simulink model "ALGO_TrajTrack_Qband"  (R2023a)
settings: Solver=VariableStepAuto  StartTime=0.0  StopTime=60  RelTol=1e-3
StopFcn:
  | CompareSimResult_anti_rollover
libraries: simulink x7, slpidlib x1, Solver_SF x1
(part 1 of 2)
CloseFcn:
  | sp_simResult_save
settings Model: Creator=QXJ  LastModifiedBy=28303
settings SolverCC: AlgebraicLoopSolver=TrustRegion
settings DebuggingCC: UnconnectedInputMsg=warning  UnconnectedOutputMsg=warning  UnconnectedLineMsg=warning
settings ModelReferenceCC: EnableRefExpFcnMdlSchedulingChecks=on
settings SFSimCC: CustomCodeUndefinedFunction=UseInterfaceOnly

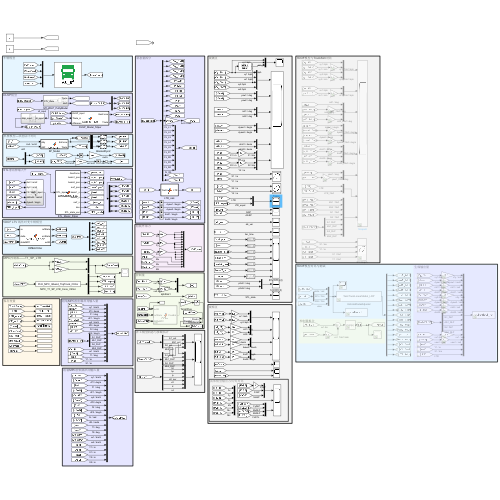
[thumbnail: Simulink's stored preview of the top-level diagram]
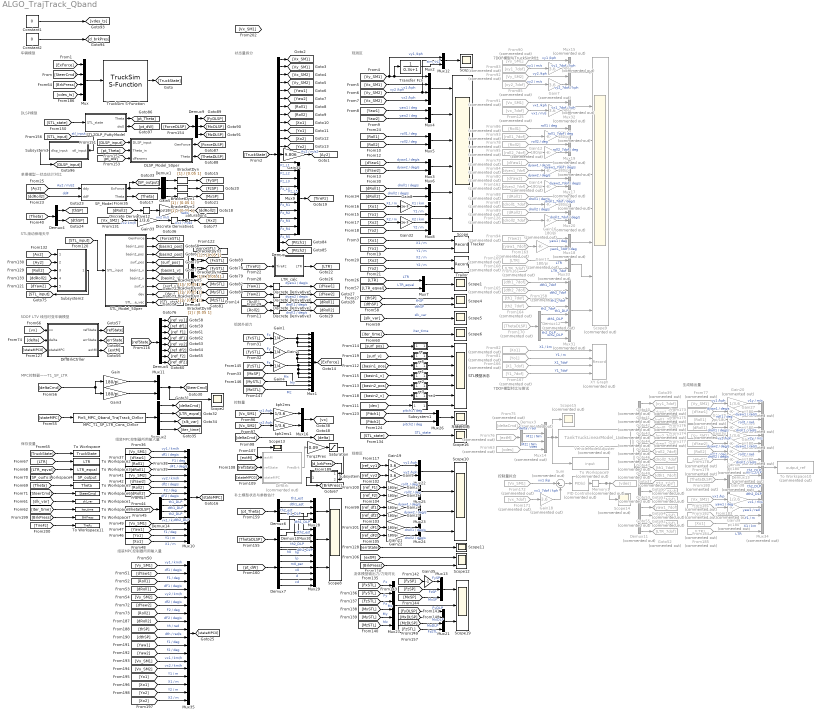
== system ALGO_TrajTrack_Qband ==
  note: 7DOF模型对比与测试
  note: 生成输出量
  note: 控制量拟合
  note: 7DOF模型与TruckSim对比
  note: 补土模型状态与参数估计
  note: 流体模型输出力/力矩对比
  note: MPC控制器——T1_SP_LTR
  note: 组装MPC控制器所用输入量
  note: 观测区
  note: 车辆模型
  note: 组装外部力
  note: 单摆模型---状态估计对比
  note: 状态量拆分
  note: 保存变量
  note: 5DOF LTV 线性时变车辆模型
  note: 观察区
  note: 控制量
  note: STL滑动伸缩天平
  note: DLSP模型
  note: 组装MPC控制器所用输入量
  BracketDyn{,1..8} (9 alike) : TransferFcn  Denominator=[0.05 1]
  Constant1 : Constant  Value=0
  Constant2 : Constant  Value=0
  DLSP_Model_50per : MATLAB Function  TreatAsAtomicUnit=on  SystemSampleTime=0.01
  Demux : Demux  Outputs=25
  Demux1 : Demux  Outputs=3
  Demux{2,6,10,14} (4 alike) : Demux
  Demux11 : Demux  Commented=on  Outputs=17
  Demux12 : Demux  Commented=on
  Demux13 : Demux  Commented=on
  Demux3 : Demux  Commented=on  Outputs=2
  Demux4 : Demux  Outputs=2
  Demux5 : Demux  Outputs=8
  Demux7 : Demux  Outputs=7
  Demux8 : Demux  Outputs=6
  Demux9 : Demux  Outputs=3
  DiffBrk : MATLAB Function  Commented=on  TreatAsAtomicUnit=on
  DiffBrkCtrller : MATLAB Function  TreatAsAtomicUnit=on  SystemSampleTime=0.01
  Discrete Derivative1 : simulink/Discrete/Discrete Derivative  gainval=1.0  ICPrevScaledInput=0  OutMin=[-9.806*0.6]  OutMax=[9.806*0.6]  OutDataType=fixdt(1, 16)  OutScaling=2^-10  DoSatur=off
  Discrete Derivative{2..3,5..6,12} (5 alike) : simulink/Discrete/Discrete Derivative  gainval=1.0  ICPrevScaledInput=0.0  OutMin=[]  OutMax=[]  OutDataType=fixdt(1, 16)  OutScaling=2^-10  DoSatur=off
  From125 : From  Commented=on  GotoTag=vx_7dof
  From126 : From  Commented=on  GotoTag=droll2_7dof
  From158 : From  Commented=on  GotoTag=th1_7dof
  From161 : From  Commented=on  GotoTag=dth1_7dof
  From162 : From  Commented=on  GotoTag=dyaw2_7dof
  From163 : From  Commented=on  GotoTag=yaw1_7dof
  From164 : From  Commented=on  GotoTag=th2_7dof
  From165 : From  Commented=on  GotoTag=dth2_7dof
  From166 : From  Commented=on  GotoTag=X1_7dof
  From167 : From  Commented=on  GotoTag=Y1_7dof
  From168 : From  Commented=on  GotoTag=LTR_7dof
  From169 : From  Commented=on  GotoTag=LTR
  From170 : From  Commented=on  GotoTag=ThetaDLSP
  From171 : From  Commented=on  GotoTag=vx_7dof
  From172 : From  Commented=on  GotoTag=Vx_SM1
  From173 : From  Commented=on  GotoTag=dYaw1
  From174 : From  Commented=on  GotoTag=Vy_SM2
  From175 : From  Commented=on  GotoTag=Roll1
  From176 : From  Commented=on  GotoTag=dRoll1
  From177 : From  Commented=on  GotoTag=dYaw2
  From178 : From  Commented=on  GotoTag=Roll2
  From179 : From  Commented=on  GotoTag=dRoll2
  From180 : From  Commented=on  GotoTag=ThetaDLSP
  From181 : From  Commented=on  GotoTag=Vx_SM1
  From182 : From  Commented=on  GotoTag=Yaw1
  From183 : From  Commented=on  GotoTag=Yo1
  From184 : From  Commented=on  GotoTag=Xo1
  From185 : From  Commented=on  GotoTag=LTR
  From63 : From  Commented=on  GotoTag=vdes
  From75 : From  Commented=on  GotoTag=deltaCmd
  From76 : From  Commented=on  GotoTag=extM
  From77 : From  Commented=on  GotoTag=Vy_SM1
  From78 : From  Commented=on  GotoTag=Roll2
  From79 : From  Commented=on  GotoTag=dYaw1
  From80 : From  Commented=on  GotoTag=dYaw2
  From81 : From  Commented=on  GotoTag=Yo1
  From82 : From  Commented=on  GotoTag=Xo1
  From83 : From  Commented=on  GotoTag=vy1_7dof
  From84 : From  Commented=on  GotoTag=dyaw1_7dof
  From85 : From  Commented=on  GotoTag=vy2_7dof
  From86 : From  Commented=on  GotoTag=Roll1
  From87 : From  Commented=on  GotoTag=droll1_7dof
  From88 : From  Commented=on  GotoTag=dRoll1
  From89 : From  Commented=on  GotoTag=dRoll2
  From90 : From  Commented=on  GotoTag=Vy_SM1
  From91 : From  Commented=on  GotoTag=Vx_SM1
  From92 : From  Commented=on  GotoTag=Vy_SM2
  From93 : From  Commented=on  GotoTag=roll1_7dof
  From94 : From  Commented=on  GotoTag=Yaw1
  From95 : From  Commented=on  GotoTag=roll2_7dof
  Gain{,3,21..26} (8 alike) : Gain  Gain=180/pi
  Gain1 : Gain  Gain=1/4
  Gain{6..7,10,18} (4 alike) : Gain  Commented=on  Gain=3.6
  Gain{11..17} (7 alike) : Gain  Commented=on  Gain=180/pi
  Gain19 : Gain  Gain=3.6
  Gain2 : Gain  Gain=1/4
  Gain20 : Gain  Commented=on  Gain=1/3.6
  Gain{27..29,31,36..37,39} (7 alike) : Gain  Commented=on  Gain=pi/180
  Gain30 : Gain  Commented=on  Gain=1/3.6
  Gain32 : Gain  Gain=1e-3
  Gain33 : Gain  Gain=1/3.6
  Gain34 : Gain  Gain=9.806
  Gain35 : Gain  Gain=-1
  Gain38 : Gain  Commented=on  Gain=1/3.6
  Gain4 : Gain  Gain=1/4
  Gain5 : Gain  Gain=pi/180
  Gain8 : Gain  Gain=1e-3
  Gain9 : Gain  Gain=3.6
  Goto37 : Goto  Commented=on  GotoTag=vdes
  Goto39 : Goto  Commented=on  GotoTag=vy1_7dof
  Goto40 : Goto  Commented=on  GotoTag=dyaw1_7dof
  Goto41 : Goto  Commented=on  GotoTag=roll1_7dof
  Goto42 : Goto  Commented=on  GotoTag=droll1_7dof
  Goto43 : Goto  Commented=on  GotoTag=vy2_7dof
  Goto44 : Goto  Commented=on  GotoTag=dyaw2_7dof
  Goto45 : Goto  Commented=on  GotoTag=roll2_7dof
  Goto46 : Goto  Commented=on  GotoTag=droll2_7dof
  Goto47 : Goto  Commented=on  GotoTag=th1_7dof
  Goto49 : Goto  Commented=on  GotoTag=dth1_7dof
  Goto50 : Goto  Commented=on  GotoTag=th2_7dof
  Goto51 : Goto  Commented=on  GotoTag=dth2_7dof
  Goto52 : Goto  Commented=on  GotoTag=LTR_7dof
  Goto53 : Goto  Commented=on  GotoTag=vx_7dof
  Goto54 : Goto  Commented=on  GotoTag=yaw1_7dof
  Goto55 : Goto  Commented=on  GotoTag=X1_7dof
  Goto92 : Goto  Commented=on  GotoTag=Y1_7dof
  "LTR_calc " : MATLAB Function  TreatAsAtomicUnit=on
  MPC_T1_SP_LTR_Cons_Ctrllor : S-Function  FunctionName=Pin5_MPC_Qband_TrajTrack_Ctrllor  SFunctionDeploymentMode=off  EnableBusSupport=off
  Memory1 : Memory  Commented=on  InitialCondition=70/3.6
  Mux{,2,8,21,28,30} (6 alike) : Mux
  Mux1 : Mux  Inputs=15
  Mux10 : Mux  Inputs=16
  Mux{3..7,11,16,22..26} (12 alike) : Mux  Inputs=2
  Mux12 : Mux  Inputs=3
  Mux13 : Mux  Inputs=3
  Mux{14..15,17,19..20} (5 alike) : Mux  Commented=on
  Mux18 : Mux  Commented=on  Inputs=2
  Mux27 : Mux  Inputs=6
  Mux29 : Mux  Inputs=7
  Mux31 : Mux  Commented=on  Inputs=8
  Mux32 : Mux  Commented=on  Inputs=2
  Mux33 : Mux  Commented=on  Inputs=2
  Mux34 : Mux  Commented=on  Inputs=17
  Mux35 : Mux  Inputs=18
  Mux9 : Mux  Inputs=10
  PID Controller : slpidlib/PID Controller  Commented=on  Controller=PID  Form=Parallel  TimeDomain=Continuous-time  UseExternalTs=off  SampleTime=-1  IntegratorMethod=Forward Euler  FilterMethod=Forward Euler  ControllerParametersSource=internal  P=5  I=5  UseKiTs=off  D=0  N=100  UseFilter=on  TunerSelectOption=Transfer Function Based (PID Tuner App)  InitialConditionSource=internal  InitialConditionForIntegrator=20  InitialConditionForFilter=0  DifferentiatorICPrevScaledInput=0  ExternalReset=none  TrackingMode=off  Kt=1  LimitOutput=off  SatLimitsSource=internal  UpperSaturationLimit=inf  LowerSaturationLimit=-inf  LinearizeAsGain=on  AntiWindupMode=none  Kb=1  LimitIntegrator=off  UpperIntegratorSaturationLimit=inf  LowerIntegratorSaturationLimit=-inf  POutMin=[]  POutMax=[]  IOutMin=[]  IOutMax=[]  DOutMin=[]  DOutMax=[]  NOutMin=[]  NOutMax=[]  SumOutMin=[]  SumOutMax=[]  SaturationOutMin=[]  SaturationOutMax=[]  PParamMin=[]  PParamMax=[]  IParamMin=[]  IParamMax=[]  DParamMin=[]  DParamMax=[]  NParamMin=[]  NParamMax=[]  KbParamMin=[]  KbParamMax=[]  KtParamMin=[]  KtParamMax=[]  KbOutMin=[]  KbOutMax=[]  KtOutMin=[]  KtOutMax=[]  IntegratorOutMin=[]  IntegratorOutMax=[]  FilterOutMin=[]  FilterOutMax=[]  SumI1OutMin=[]  SumI1OutMax=[]  SumI2OutMin=[]  SumI2OutMax=[]  SumI3OutMin=[]  SumI3OutMax=[]  SumI4OutMin=[]  SumI4OutMax=[]  SumDOutMin=[]  SumDOutMax=[]  DifferentiatorOutMin=[]  DifferentiatorOutMax=[]  FilterDiffOutCoefMin=[]  FilterDiffOutCoefMax=[]  ReciprocalOutMin=[]  ReciprocalOutMax=[]  SumDenOutMin=[]  SumDenOutMax=[]  SumNumOutMin=[]  SumNumOutMax=[]  DivideOutMin=[]  DivideOutMax=[]  UdiffTsProdOutMin=[]  UdiffTsProdOutMax=[]  NTsProdOutMin=[]  NTsProdOutMax=[]  UintegralTsProdOutMin=[]  UintegralTsProdOutMax=[]  UngainTsProdOutMin=[]  UngainTsProdOutMax=[]  ClampingZeroOutDataTypeStr=Inherit: Inherit via back propagation  ClampingZeroOutMin=[]  ClampingZeroOutMax=[]  FilterDenConstantOutDataTypeStr=Inherit: Inherit via back propagation  FilterDenConstantOutMin=[]  FilterDenConstantOutMax=[]  PCopyOutDataTypeStr=Inherit: Inherit via back propagation  PCopyOutMin=[]  PCopyOutMax=[]  NCopyOutDataTypeStr=Inherit: Inherit via back propagation  NCopyOutMin=[]  NCopyOutMax=[]  IntegratorContinuousStateAttributes=''  IntegratorStateMustResolveToSignalObject=off  IntegratorRTWStateStorageClass=Auto  FilterContinuousStateAttributes=''  FilterStateMustResolveToSignalObject=off  FilterRTWStateStorageClass=Auto  ParallelPVariant=InternalParameters  IdealPVariant=Disabled  IVariant=InternalParameters  DVariant=InternalParameters  IntegratorVariant=Continuous  SatVariant=Disabled  AWVariant=Passthrough  PCopyVariant=Disabled  TRVariant=Disabled  FdbkBlocksVariant=Forward  IdealPFdbkVariant=Disabled  SatFdbkVariant=Disabled  DerivativeFilterVariant=ContFilter  NVariant=InternalParameters  NCopyVariant=Disabled  FilterICVariant=InternalICsFilter  IntegratorICVariant=InternalICs  ExternalResetVariant=Disabled  TRSumVariant=Passthrough  SumFdbkVariant=Disabled  SumVariant=Sum_PID  TsampFilterVariant=InternalTs  TsampNgainVariant=Passthrough  TsampIntegralVariant=Disabled_SignalSpec  ExternalSaturationOutDataTypeStr=Inherit: Same as second input
  SP_Model : MATLAB Function  TreatAsAtomicUnit=on  SystemSampleTime=0.005
  STL2DLP_PuttyModel : Subsystem
  STL_Model_50per : MATLAB Function  TreatAsAtomicUnit=on  SystemSampleTime=0.01
  STL模型状态 : Scope  NumInputPorts=7
  Saturation : Saturate  UpperLimit=0.75  LowerLimit=0
  Saturation1 : Saturate  UpperLimit=9.806*0.6  LowerLimit=-9.806*0.6
  Scope : Scope  NumInputPorts=6
  Scope{1..3,5..6,11,13,16} (8 alike) : Scope
  Scope10 : Scope  NumInputPorts=4
  Scope12 : Scope  NumInputPorts=2
  Scope14 : Scope  Commented=on
  Scope15 : Scope  Commented=on
  Scope19 : Scope  NumInputPorts=3
  Scope4 : Scope  NumInputPorts=2
  Scope8 : Scope  NumInputPorts=3
  Scope9 : Scope  Commented=on  NumInputPorts=8
  Subsystem : Subsystem
  Subsystem1 : Subsystem
  Subsystem2 : Subsystem
  Subsystem3 : Subsystem
  Sum : Sum  Commented=on  Inputs=|+-
  To Workspace : ToWorkspace  VariableName=TruckState  SaveFormat=Timeseries  SampleTime=-1
  To Workspace1 : ToWorkspace  VariableName=skl_var  SaveFormat=Timeseries  SampleTime=-1
  To Workspace10 : ToWorkspace  Commented=on  VariableName=output_ref  SaveFormat=Timeseries  SampleTime=-1
  To Workspace11 : ToWorkspace  VariableName=TireFz  SaveFormat=Timeseries  SampleTime=-1
  To Workspace2 : ToWorkspace  VariableName=LTR  SaveFormat=Timeseries  SampleTime=-1
  To Workspace3 : ToWorkspace  VariableName=LTR_eqval  SaveFormat=Timeseries  SampleTime=-1
  To Workspace4 : ToWorkspace  VariableName=SP_output  SaveFormat=Timeseries  SampleTime=-1
  To Workspace5 : ToWorkspace  VariableName=Theta  SaveFormat=Timeseries  SampleTime=-1
  To Workspace6 : ToWorkspace  VariableName=SteerCmd  SaveFormat=Timeseries  SampleTime=-1
  To Workspace7 : ToWorkspace  VariableName=BrkPress  SaveFormat=Timeseries  SampleTime=-1
  To Workspace8 : ToWorkspace  VariableName=iter_time  SaveFormat=Timeseries  SampleTime=-1
  To Workspace9 : ToWorkspace  Commented=on  VariableName=input  SaveFormat=Timeseries  SampleTime=-1
  Torq2Pres : Gain  Gain=0.09
  Tracker : Record  FileSettingsInternal="{\"entries\":[{\"content\":{\"excelSettings\":{\"content\":{},\"type\":\"Streamout.ExcelSettings\"}},\"type\":\"Streamout.FileSettingStorage\",\"uuid\":\"10e10eac-3b42-48c4-b005-3ff0f1f86fec\"}],\"packageUris\":[\"http://schema.mathworks.com/mf0/streamout_blocks/R2020a\"],\"version\":\"1.0\"}"  Layout=[1 1]  SignalsInternal="{\"entries\":[{\"content\":{\"signals\":[{\"content\":{\"blockPath\":[\"ALGO_TrajTrack_Qband/Tracker\"],\"dimensions\":[1],\"domain\":\"ALGO_TrajTrack_Qband/Tracker\",\"lineColor\":\"#64d413\",\"port\":1,\"sid\":[\"\"],\"signalID\":23696,\"signalName\":\"X1 / m\"},\"type\":\"RecordBlkView.Signal\",\"uuid\":\"81066948-288f-4e97-bbd3-45679b52fbb6\"},{\"content\":{\"blockPath\":[\"ALGO_TrajTrack_Qband/Tracker\"],\"dimensions\":[1],\"domain\":\"ALGO_TrajTrack_Qband/Tracker\",\"lineColor\":\"#ff13a6\",\"port\":2,\"sid\":[\"\"],\"signalID\":23700,\"signalName\":\"Y1 / m\"},\"type\":\"RecordBlkView.Signal\",\"uuid\":\"ec9d7904-73b7-4926-97ce-8ccb334fc86a\"}]},\"type\":\"RecordBlkView.InputSignals\",\"uuid\":\"48fa4a27-7477-4a7c-bc50-316526f17c74\"}],\"packageUris\":[\"http://schema.mathworks.com/mf0/streamout_blocks/R2020a\"],\"version\":\"1.0\"}"  VisualizationBindings="{\"xyplotplugin\":{\"info\":[{\"series\":[],\"subplotID\":1}]}}"  CompatibilityTag=XY  st=-1
  "Trailor " : Record  FileSettingsInternal="{\"entries\":[{\"content\":{\"excelSettings\":{\"content\":{},\"type\":\"Streamout.ExcelSettings\"}},\"type\":\"Streamout.FileSettingStorage\",\"uuid\":\"faa460d8-38ba-47e0-98d6-491682c65f2f\"}],\"packageUris\":[\"http://schema.mathworks.com/mf0/streamout_blocks/R2020a\"],\"version\":\"1.0\"}"  Layout=[1 1]  SignalsInternal="{\"entries\":[{\"content\":{\"signals\":[{\"content\":{\"blockPath\":[\"ALGO_TrajTrack_Qband/Trailor \"],\"dimensions\":[1],\"domain\":\"ALGO_TrajTrack_Qband/Trailor \",\"lineColor\":\"#fe330a\",\"port\":1,\"sid\":[\"\"],\"signalID\":23704,\"signalName\":\"X2 / m\"},\"type\":\"RecordBlkView.Signal\",\"uuid\":\"b72d44ec-ecbc-4ebd-8289-1d930c6df7ac\"},{\"content\":{\"blockPath\":[\"ALGO_TrajTrack_Qband/Trailor \"],\"dimensions\":[1],\"domain\":\"ALGO_TrajTrack_Qband/Trailor \",\"lineColor\":\"#22b573\",\"port\":2,\"sid\":[\"\"],\"signalID\":23708,\"signalName\":\"Y2 / m\"},\"type\":\"RecordBlkView.Signal\",\"uuid\":\"1ebb3757-e1f8-4087-92ac-93cb986b12b2\"}]},\"type\":\"RecordBlkView.InputSignals\",\"uuid\":\"6de3b5d5-cdc3-4095-8524-c1b517bba064\"}],\"packageUris\":[\"http://schema.mathworks.com/mf0/streamout_blocks/R2020a\"],\"version\":\"1.0\"}"  VisualizationBindings="{\"xyplotplugin\":{\"info\":[{\"series\":[],\"subplotID\":1}]}}"  CompatibilityTag=XY  st=-1
  Transfer Fcn : TransferFcn  Denominator=[0.3 1]
  TruckSim S-Function : Solver_SF/TruckSim S-Function  Priority=1  SIMFILE=ALGO_Tanker_TrajTrack_Qband.sim
      settings: SourceProductName=TruckSim S-Function
  VehicleModelAdjuster : S-Function  Commented=on  FunctionName=TankTruckLinearModel_LDP  SFunctionDeploymentMode=off  EnableBusSupport=off
  XY Graph : Record  Commented=on  FileSettingsInternal="{\"entries\":[{\"content\":{\"excelSettings\":{\"content\":{},\"type\":\"Streamout.ExcelSettings\"}},\"type\":\"Streamout.FileSettingStorage\",\"uuid\":\"db5158d0-9919-4d7c-8365-e16bcbc2540d\"}],\"packageUris\":[\"http://schema.mathworks.com/mf0/streamout_blocks/R2020a\"],\"version\":\"1.0\"}"  Layout=[1 1]  SignalsInternal="{\"entries\":[{\"content\":{},\"type\":\"RecordBlkView.InputSignals\",\"uuid\":\"bb9bc6a2-9b99-4422-9b16-66f0088ca28f\"}],\"packageUris\":[\"http://schema.mathworks.com/mf0/streamout_blocks/R2020a\"],\"version\":\"1.0\"}"  VisualizationBindings="{\"xyplotplugin\":{\"info\":[{\"series\":[],\"subplotID\":1}]}}"  CompatibilityTag=XY
  kph2ms : Gain  Gain=1/3.6
  kph2ms1 : Gain  Gain=1/3.6
  re : Subsystem
  re1 : Subsystem
  re2 : Subsystem
  re3 : Subsystem
  re4 : Subsystem
  re5 : Subsystem
  车辆俯仰角 : Scope
  wires:
  TruckSim S-Function/1 -> [TruckState]
  Mux/1 -> TruckSim S-Function/1
  Discrete Derivative12/1 -> Gain5/1
  Demux4/2 -> [dthSP]
  Demux4/1 -> [thSP]
  [Theta] -> Demux4/1
  [Ay2] -> SP_Model/1(ddy)  "Ay2 / m/s2"
  Gain5/1 -> [ddRoll2]  "rad/s"
  Gain2/1 -> Mux1/8, Mux1/7, Mux1/6, Mux1/5
  Gain1/1 -> Mux1/4, Mux1/3, Mux1/2, Mux1/1
  [dRoll2] -> Discrete Derivative12/1
  [ddRoll2] -> SP_Model/2(ddF)  "ddF"
  BracketDyn/1 -> [FySP]
  BracketDyn1/1 -> [FzSP]
  BracketDyn2/1 -> [MxSP]
  SP_Model/1(ExForce) -> Demux1/1, [SP_output]
  Demux1/1 -> BracketDyn/1
  Demux1/2 -> BracketDyn1/1
  Demux1/3 -> BracketDyn2/1
  SP_Model/2(Theta) -> [Theta]
  Mux1/1 -> [ExForce]
  [Yo1] -> Mux8/2  "Y1 / m"
  [Roll1] -> Mux5/1  "roll1 / deg"
  Mux3/1 -> Scope/4
  [Vx_SM1] -> Mux2/2  "vx1 /kph"
  [dRoll1] -> Mux6/1  "droll1 / deg/s"
  [Xo1] -> Tracker/1  "X1 / m"
  [Roll2] -> Mux5/2  "roll2 / deg"
  Mux8/1 -> Scope/6
  [Yo1] -> Tracker/2  "Y1 / m"
  Mux6/1 -> Scope/5
  Mux2/1 -> Scope/1
  [Yo2] -> "Trailor "/2  "Y2 / m"
  [dYaw2] -> Mux3/2  "dyaw2 / deg/s"
  [Yaw2] -> Mux4/2  "yaw2 / deg"
  [Vx_SM2] -> Mux2/4  "vx2 /kph"
  Mux5/1 -> Scope/3
  [Xo1] -> Gain8/1  "X1 / m"
  [Yaw1] -> Mux4/1  "yaw1 / deg"
  [Vy_SM2] -> Mux12/2, Mux2/3  "vy2 /kph"
  [dYaw1] -> Mux3/1  "dyaw1 / deg/s"
  [Yo2] -> Mux8/4  "Y2 / m"
  Mux4/1 -> Scope/2
  [Xo2] -> Gain32/1  "X2 / m"
  [Xo2] -> "Trailor "/1  "X2 / m"
  [Vy_SM1] -> Mux12/1, Transfer Fcn/1, Mux2/1  "vy1 /kph"
  [dRoll2] -> Mux6/2  "droll2 / deg/s"
  Demux/13 -> Gain34/1
  Demux/8 -> [Roll2]
  Demux/6 -> [Yaw2]
  Demux/2 -> [Vy_SM1]
  Demux/4 -> [Vy_SM2]
  Demux/9 -> [Xo1]
  Demux/10 -> [Yo1]
  Demux/11 -> [Xo2]
  Demux/7 -> [Roll1]
  Demux/5 -> [Yaw1]
  Demux/1 -> [Vx_SM1]
  Demux/3 -> [Vx_SM2]
  Demux/12 -> [Yo2]
  [TruckState] -> Demux/1
  Demux/14 -> Mux9/1  "Fz_L1"
  Demux/15 -> Mux9/2  "Fz_L2"
  Demux/16 -> Mux9/3  "Fz_L3"
  Demux/17 -> Mux9/4  "Fz_L4"
  Demux/18 -> Mux9/5  "Fz_L5"
  Demux/19 -> Mux9/6  "Fz_R1"
  Demux/20 -> Mux9/7  "Fz_R2"
  Demux/21 -> Mux9/8  "Fz_R3"
  Demux/22 -> Mux9/9  "Fz_R4"
  Demux/23 -> Mux9/10  "Fz_R5"
  Mux9/1 -> [TireFz]
  [TireFz] -> "LTR_calc "/1(TireFz)
  "LTR_calc "/1(LTR) -> [LTR]
  [Yaw2] -> Discrete Derivative6/1
  Discrete Derivative5/1 -> [dYaw1]  "dyaw1 / deg/s"
  [Yaw1] -> Discrete Derivative5/1
  Discrete Derivative6/1 -> [dYaw2]  "dyaw2 / deg/s"
  [Roll1] -> Discrete Derivative2/1
  [Roll2] -> Discrete Derivative3/1
  Discrete Derivative2/1 -> [dRoll1]  "droll1 / deg/s"
  Discrete Derivative3/1 -> [dRoll2]  "droll2 / deg/s"
  [ExForce] -> Mux/1
  [SteerCmd] -> Mux/2
  [Vy_SM1] -> Mux10/1  "vy1 / km/h"
  [dYaw1] -> Mux10/2  "df1 / deg/s"
  [Roll1] -> Mux10/3  "F1 / deg"
  [dRoll1] -> Mux10/4  "dF1 / deg/s"
  [Vy_SM2] -> Mux10/5  "vy2 / km/h"
  [dYaw2] -> Mux10/6  "df2 / deg/s"
  [Roll2] -> Mux10/7  "F2 / deg"
  [dRoll2] -> Mux10/8  "dF2 / deg/s"
  [Yaw1] -> Mux10/14  "f1 / deg"
  [Vx_SM1] -> Mux10/13  "vx1 / km/h"
  Mux10/1 -> [stateMPC]
  [stateMPC] -> MPC_T1_SP_LTR_Cons_Ctrllor/1
  Mux11/1 -> Scope2/1, [SteerCmd]
  Gain/1 -> Mux11/1
  Gain3/1 -> Mux11/2
  [LTR] -> Mux7/1  "LTR"
  [LTR_eqval] -> Mux7/2  "LTR_eqval"
  Mux7/1 -> Scope1/1
  [iter_time] -> To Workspace8/1
  [iter_time] -> Scope6/1  "iter_time"
  [SP_output] -> To Workspace4/1
  [slk_var] -> Scope5/1  "slk_var"
  [Theta] -> To Workspace5/1
  [TruckState] -> To Workspace/1
  [LTR_eqval] -> To Workspace3/1
  [slk_var] -> To Workspace1/1
  [SteerCmd] -> To Workspace6/1
  [LTR] -> To Workspace2/1
  [thSP] -> Scope4/1  "thSP"
  [dthSP] -> Scope4/2  "dthSP"
  Demux2/2 -> [LTR_eqval]
  Demux2/1 -> [deltaCmd]
  MPC_T1_SP_LTR_Cons_Ctrllor/1 -> Demux2/1
  Transfer Fcn/1 -> Mux12/3  "sim_vy2"
  Mux12/1 -> Scope3/1
  Gain35/1 -> Mux13/1  "FySP"
  [FzSP] -> Mux13/2  "FzSP"
  [MxSP] -> Mux13/3  "MxSP"
  Mux13/1 -> Scope19/1
  [ref_F1] -> Gain25/1
  [refState] -> Demux5/1
  Demux5/2 -> [ref_df1]
  [errState] -> Scope11/1
  Gain21/1 -> Mux24/1  "droll1 / deg/s"
  Gain22/1 -> Mux24/2  "droll2 / deg/s"
  [Vx_SM2] -> kph2ms1/1  "vx2 /kph"
  Demux5/1 -> [ref_vy1]
  [Vx_SM1] -> kph2ms/1  "vx1 /kph"
  [deltaCmd] -> [delta]
  [extM] -> Scope13/1, DiffBrk/1(extM)
  Demux5/4 -> [ref_dF1]
  [stateMPC0] -> DiffBrkCtrller/3(stateMPC)
  [stateMPC0] -> DiffBrk/3(stateMPC)
  DiffBrk/1(PresBrk) -> Torq2Pres/1
  Demux5/5 -> [ref_vy2]
  Gain26/1 -> Mux25/2  "roll2 / deg"
  Mux23/1 -> Scope10/3
  [ref_F2] -> Gain26/1
  [ref_df2] -> Gain23/1
  Saturation/1 -> Subsystem/1(PresIn)
  [refState] -> DiffBrk/2(refState)
  Demux5/3 -> [ref_F1]
  [BrkPress] -> Scope12/2
  Gain19/1 -> Mux22/1  "vy1 /kph"
  [extM] -> Scope12/1
  Gain9/1 -> Mux22/2  "vy2 /kph"
  Mux16/1 -> [vx]
  Gain25/1 -> Mux25/1  "roll1 / deg"
  [ref_dF1] -> Gain21/1
  DiffBrkCtrller/2(errState) -> [errState]
  [ref_dF2] -> Gain22/1
  DiffBrkCtrller/3(extM) -> [extM]
  Mux25/1 -> Scope10/2
  [ref_vy1] -> Gain19/1
  Mux24/1 -> Scope10/4
  kph2ms1/1 -> Mux16/2
  Mux22/1 -> Scope10/1
  Demux5/8 -> [ref_dF2]
  Demux5/7 -> [ref_F2]
  Gain23/1 -> Mux23/2  "dyaw2 / deg/s"
  DiffBrkCtrller/1(refState) -> [refState]
  Demux5/6 -> [ref_df2]
  [vx] -> DiffBrkCtrller/1(vx)
  Gain24/1 -> Mux23/1  "dyaw1 / deg/s"
  kph2ms/1 -> Mux16/1
  [ref_df1] -> Gain24/1
  [delta] -> DiffBrkCtrller/2(delta)
  [ref_vy2] -> Gain9/1
  Subsystem/1(PresOut) -> [BrkPress]
  [BrkPress] -> Mux/3
  [surf_pos] -> re/1(In1)
  re/1(Out1) -> STL模型状态/1
  re2/1(Out1) -> STL模型状态/4
  re5/1(Out1) -> STL模型状态/2
  [basin1_v] -> re2/1(In1)
  [surf_v] -> re5/1(In1)
  [basin2_v] -> re4/1(In1)
  [basin2_pos] -> re3/1(In1)
  re4/1(Out1) -> STL模型状态/6
  Subsystem1/1(Out1) -> STL模型状态/7
  [dev] -> Subsystem1/1(In1)
  re1/1(Out1) -> STL模型状态/3
  [basin1_pos] -> re1/1(In1)
  re3/1(Out1) -> STL模型状态/5
  STL_Model_50per/5(basin1_v) -> [basin1_v]
  STL_Model_50per/1(GenForce) -> [ForceSTL]
  STL_Model_50per/9(STL_state_vec) -> [STL_state]
  STL_Model_50per/3(basin2_pos) -> [basin2_pos]
  [STL_input] -> STL_Model_50per/1(STL_input)
  STL_Model_50per/6(basin2_v) -> [basin2_v]
  STL_Model_50per/2(basin1_pos) -> [basin1_pos]
  STL_Model_50per/8(dev) -> [dev]
  STL_Model_50per/4(surf_pos) -> [surf_pos]
  STL_Model_50per/7(surf_v) -> [surf_v]
  [Vx_SM2] -> Gain33/1  "vx2 km/h"
  Gain33/1 -> Discrete Derivative1/1  "vx2 m/s"
  Discrete Derivative1/1 -> Saturation1/1  "Ax2 / m/s2"
  Gain34/1 -> [Ay2]  "Ay2 / m/s2"
  Demux8/2 -> BracketDyn4/1
  Demux8/3 -> BracketDyn5/1
  [ForceSTL] -> Demux8/1
  Demux8/6 -> BracketDyn8/1
  Demux8/4 -> BracketDyn6/1
  Demux8/1 -> BracketDyn3/1
  Demux8/5 -> BracketDyn7/1
  Demux/24 -> [Pitch1]
  Demux/25 -> [Pitch2]
  Mux26/1 -> 车辆俯仰角/1
  [Pitch1] -> Mux26/1  "pitch1 / deg"
  [Pitch2] -> Mux26/2  "pitch2 / deg"
  [STL_state] -> Scope16/1  "STL_state"
  Mux27/1 -> Scope19/2
  Saturation1/1 -> [Ax2]
  [MySTL] -> Mux27/5  "My"
  [MzSTL] -> Mux27/6  "Mz"
  BracketDyn3/1 -> [FxSTL]
  BracketDyn4/1 -> [FySTL]
  BracketDyn5/1 -> [FzSTL]
  BracketDyn6/1 -> [MxSTL]
  BracketDyn7/1 -> [MySTL]
  BracketDyn8/1 -> [MzSTL]
  [FySP] -> Gain35/1
  [FxSTL] -> Gain1/1  "Fx"
  [FySTL] -> Gain2/1  "Fy"
  [FzSTL] -> Gain4/1  "Fz"
  Gain4/1 -> Mux1/12, Mux1/11, Mux1/10, Mux1/9
  [MySTL] -> Mux1/14  "My"
  [Ax2] -> Subsystem2/1(Ax2 / m/s2)
  [Ay2] -> Subsystem2/2(Ay2 / m/s2)
  [Roll2] -> Subsystem2/3(F2 / deg)
  [ddRoll2] -> Subsystem2/4(ddRoll2 / rad/s2)
  [dYaw2] -> Subsystem2/5(dyaw2 / deg/s)
  Subsystem2/1(STL_input) -> [STL_input]
  [MzSTL] -> Mux1/15  "Mz"
  [MxSP] -> Mux1/13  "Mx"
  Gain8/1 -> Mux8/1  "X1 / km"
  Gain32/1 -> Mux8/3  "X2 / km"
  [pt_Theta] -> DLSP_Model_50per/2(Theta_in)
  DLSP_Model_50per/1(GenForce) -> [ForceDLSP]
  [DLSP_input] -> DLSP_Model_50per/1(DLSP_input)
  [pt_dW] -> DLSP_Model_50per/3(dParams)
  DLSP_Model_50per/2(Theta) -> [ThetaDLSP]
  Demux9/2 -> [MxDLSP]
  Demux9/3 -> [MzDLSP]
  [ForceDLSP] -> Demux9/1
  Demux9/1 -> [FyDLSP]
  [STL_input] -> Subsystem3/1(stl_input)  "stl_input"
  Subsystem3/1(dlsp_input) -> [DLSP_input]
  [MxDLSP] -> Mux21/2  "MxDLP"
  [MzDLSP] -> Mux21/3  "MzDLP"
  [FyDLSP] -> Mux21/1  "FyDLP"
  Mux21/1 -> Scope19/3
  Torq2Pres/1 -> Saturation/1
  Demux7/2 -> Mux29/2  "hp"
  Mux28/1 -> Scope8/1
  Demux6/1 -> Mux28/1  "th1_est"
  Demux6/2 -> Mux28/2  "dth1_est"
  Demux7/3 -> Mux29/3  "lp"
  Demux7/1 -> Mux29/1  "h0"
  Demux7/5 -> Mux29/5  "x0"
  Demux7/6 -> Mux29/6  "d"
  Demux7/4 -> Mux29/4  "m0_per"
  Mux29/1 -> Scope8/3
  Demux7/7 -> Mux29/7  "cd"
  [pt_Theta] -> Demux6/1
  [pt_dW] -> Demux7/1
  [FxSTL] -> Mux27/1  "Fx"
  [FySTL] -> Mux27/2  "Fy"
  [FzSTL] -> Mux27/3  "Fz"
  [MxSTL] -> Mux27/4  "Mx"
  [STL_state] -> STL2DLP_PuttyModel/1(STL_state)
  STL2DLP_PuttyModel/2(dw0) -> [pt_dW]
  STL2DLP_PuttyModel/1(Theta) -> [pt_Theta]
  [ThetaDLSP] -> Demux10/1
  Demux10/1 -> Mux28/3  "th1_DLP"
  Demux10/2 -> Mux28/4  "dth1_DLP"
  Demux6/3 -> Mux30/1  "th2_est"
  Demux6/4 -> Mux30/2  "dth2_est"
  Demux10/3 -> Mux30/3  "th2_DLP"
  Demux10/4 -> Mux30/4  "dth2_DLP"
  Mux30/1 -> Scope8/2
  [FzSTL] -> Mux21/4  "FzSTL"
  From63/1 -> Mux14/4  "vdes"
  From75/1 -> Mux14/1  "delta / rad"
  From76/1 -> Demux3/1
  Demux3/1 -> Mux14/2  "M1z / Nm"
  Demux3/2 -> Mux14/3  "M2z / Nm"
  Mux14/1 -> Scope15/1, To Workspace9/1, VehicleModelAdjuster/1
  VehicleModelAdjuster/1 -> Demux11/1
  Mux19/1 -> Scope9/3
  From78/1 -> Mux19/3  "roll2 / deg"
  Mux17/1 -> Scope9/4
  From79/1 -> Mux17/1  "dyaw1 / deg/s"
  Mux15/1 -> Scope9/1
  Mux20/1 -> Scope9/5
  From86/1 -> Mux19/1  "roll1 / deg"
  From94/1 -> Mux18/1  "yaw1 / deg"
  Demux11/1 -> Goto39/1
  Demux11/2 -> Goto40/1
  Demux11/3 -> Goto41/1
  Demux11/4 -> Goto42/1
  Demux11/5 -> Goto43/1
  Demux11/6 -> Goto44/1
  Demux11/7 -> Goto45/1
  Demux11/8 -> Goto46/1
  Demux11/9 -> Goto47/1
  Demux11/10 -> Goto49/1
  Demux11/11 -> Goto50/1
  Demux11/12 -> Goto51/1
  Demux11/17 -> Goto52/1
  Demux11/13 -> Goto53/1
  Demux11/14 -> Goto54/1
  From90/1 -> Mux15/1  "vy1 /kph"
  From83/1 -> Gain6/1  "vy1 / m/s"
  From92/1 -> Mux15/3  "vy2 /kph"
  From85/1 -> Gain7/1  "vy2 / m/s"
  Mux32/1 -> Scope9/2
  From91/1 -> Mux32/1  "vx1 /kph"
  From125/1 -> Gain10/1  "vx1 / m/s"
  From84/1 -> Gain13/1
  From80/1 -> Mux17/3  "dyaw2 / deg/s"
  From162/1 -> Gain14/1
  From93/1 -> Gain11/1
  From95/1 -> Gain12/1
  From88/1 -> Mux20/1  "droll1 / deg/s"
  From87/1 -> Gain15/1
  From89/1 -> Mux20/3  "droll2 / deg/s"
  From126/1 -> Gain16/1
  From163/1 -> Gain17/1
  From169/1 -> Mux33/1  "LTR"
  From168/1 -> Mux33/2  "LTR_7dof"
  From81/1 -> XY Graph/2  "Y1 / m"
  From82/1 -> XY Graph/1  "X1 / km"
  From166/1 -> XY Graph/3  "X1_7dof"
  From167/1 -> XY Graph/4  "Y1_7dof"
  Gain7/1 -> Mux15/4  "vy2_7dof / kph"
  Gain10/1 -> Mux32/2  "vx1_7dof / kph"
  Gain11/1 -> Mux19/2  "roll1_7dof / deg"
  Gain12/1 -> Mux19/4  "roll2_7dof / deg"
  Gain13/1 -> Mux17/2  "dyaw1_7dof / deg/s"
  Gain14/1 -> Mux17/4  "dyaw2_7dof / deg/s"
  Gain15/1 -> Mux20/2  "droll1_7dof / deg/s"
  Gain16/1 -> Mux20/4  "droll2_7dof / deg/s"
  Gain17/1 -> Mux18/2  "yaw1_7dof / deg"
  Mux18/1 -> Scope9/6
  Mux33/1 -> Scope9/7
  From170/1 -> Demux12/1
  From161/1 -> Mux31/1  "dth1_7dof"
  From165/1 -> Mux31/2  "dth2_7dof"
  From158/1 -> Mux31/3  "th1_7dof"
  From164/1 -> Mux31/4  "th2_7dof"
  Demux12/4 -> Mux31/8  "dth2_DLP"
  Demux12/3 -> Mux31/7  "th2_DLP"
  Demux12/2 -> Mux31/6  "dth1_DLP"
  Demux12/1 -> Mux31/5  "th1_DLP"
  Mux31/1 -> Scope9/8
  Gain6/1 -> Mux15/2  "vy1_7dof / kph"
  Sum/1 -> PID Controller/1
  From171/1 -> Gain18/1
  From172/1 -> Sum/1  "vx1 /kp"
  Gain18/1 -> Sum/2  "vx1_7dof / kph"
  Memory1/1 -> Scope14/1, Goto37/1
  PID Controller/1 -> Memory1/1
  Demux11/15 -> Goto92/1
  Demux11/16 -> Goto55/1
  From77/1 -> Gain20/1  "vy1 /kph"
  Gain20/1 -> Mux34/1  "v1y / m/s"
  From173/1 -> Gain27/1  "dyaw1 / deg/s"
  Gain27/1 -> Mux34/2  "dyaw1 / rad/s"
  From175/1 -> Gain28/1  "roll1 / deg"
  Gain28/1 -> Mux34/3  "roll1 / rad"
  From176/1 -> Gain29/1  "droll1 / deg/s"
  Gain29/1 -> Mux34/4  "droll1 / rad/s"
  From174/1 -> Gain30/1  "vy2 /kph"
  Gain30/1 -> Mux34/5  "v2y / m/s"
  From177/1 -> Gain31/1  "dyaw2 / deg/s"
  Gain31/1 -> Mux34/6  "dyaw2 / rad/s"
  From178/1 -> Gain36/1  "roll2 / deg"
  Gain36/1 -> Mux34/7  "roll2 / rad"
  From179/1 -> Gain37/1  "droll2 / deg/s"
  Gain37/1 -> Mux34/8  "droll2 / rad/s"
  From180/1 -> Demux13/1
  Demux13/4 -> Mux34/12  "dth2_DLP"
  Demux13/3 -> Mux34/11  "th2_DLP"
  Demux13/2 -> Mux34/10  "dth1_DLP"
  Demux13/1 -> Mux34/9  "th1_DLP"
  From181/1 -> Gain38/1  "vx1 /kp"
  Gain38/1 -> Mux34/13  "vx1 / m/s"
  From182/1 -> Gain39/1  "yaw1 / deg"
  Gain39/1 -> Mux34/14  "yaw1 / rad"
  From184/1 -> Mux34/16  "X1 / km"
  From183/1 -> Mux34/15  "Y1 / m"
  From185/1 -> Mux34/17  "LTR"
  Mux34/1 -> To Workspace10/1
  [vdes_ts] -> Mux/4
  [deltaCmd] -> Gain3/1, Gain/1
  [d_brkPres] -> Subsystem/2(PresDecel)
  Constant2/1 -> [d_brkPres]
  [ThetaDLSP] -> Demux14/1
  Demux14/1 -> Mux10/9  "th1_DLP"
  Demux14/2 -> Mux10/10  "dth1_DLP"
  Demux14/3 -> Mux10/11  "th2_DLP"
  Demux14/4 -> Mux10/12  "dth2_DLP"
  Demux2/3 -> [slk_var]
  Demux2/4 -> [iter_time]
  [Yo1] -> Mux10/15  "Y1 / m"
  [Xo1] -> Mux10/16  "X1 / m"
  [Vy_SM2] -> Mux35/5  "vy2 / km/h"
  [thSP] -> Mux35/9  "th / rad"
  [dRoll1] -> Mux35/4  "dF1 / deg/s"
  [dYaw2] -> Mux35/6  "df2 / deg/s"
  [dRoll2] -> Mux35/8  "dF2 / deg/s"
  [Yaw2] -> Mux35/12  "f2 / deg"
  [Xo1] -> Mux35/16  "X1 / m"
  [Roll1] -> Mux35/3  "F1 / deg"
  [Vy_SM1] -> Mux35/1  "vy1 / km/h"
  [Yo2] -> Mux35/17  "Y2 / m"
  [Xo2] -> Mux35/18  "X2 / m"
  [Vx_SM2] -> Mux35/14  "vx2 / km/h"
  [Roll2] -> Mux35/7  "F2 / deg"
  [dYaw1] -> Mux35/2  "df1 / deg/s"
  [Yo1] -> Mux35/15  "Y1 / m"
  [Vx_SM1] -> Mux35/13  "vx1 / km/h"
  [Yaw1] -> Mux35/11  "f1 / deg"
  Mux35/1 -> [stateMPC0]
  [dthSP] -> Mux35/10  "dth / rad/s"
  [BrkPress] -> To Workspace7/1
  [TireFz] -> To Workspace11/1
  Constant1/1 -> [vdes_ts]

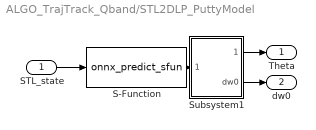
== system ALGO_TrajTrack_Qband/STL2DLP_PuttyModel ==
  STL_state : Inport
  S-Function : S-Function  FunctionName=onnx_predict_sfun  SFunctionDeploymentMode=off  EnableBusSupport=off
  Subsystem1 : Subsystem
  Theta : Outport
  dw0 : Outport  Port=2
  wires:
  S-Function/1 -> Subsystem1/1(STL_State)
  STL_state/1 -> S-Function/1
  Subsystem1/1(Theta) -> Theta/1
  Subsystem1/2(dw0) -> dw0/1

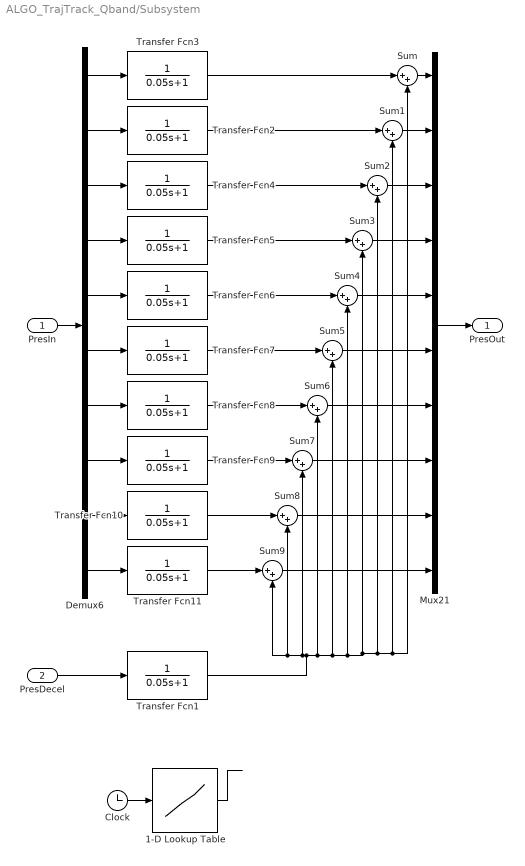
== system ALGO_TrajTrack_Qband/Subsystem ==
  PresIn : Inport
  PresDecel : Inport  Port=2
  1-D Lookup Table : Lookup_n-D  NumberOfTableDimensions=1  BreakpointsForDimension1=[0 5 6 7 15]  Table=[0 0 0.2 0 0]  InternalRulePriority=Speed  RndMeth=Simplest
  Clock : Clock
  Demux6 : Demux  Outputs=10
  Mux21 : Mux  Inputs=10
  Sum{,1..9} (10 alike) : Sum  Inputs=|++
  Transfer Fcn{1..11} (11 alike) : TransferFcn  Denominator=[0.05 1]
  PresOut : Outport
  wires:
  Demux6/10 -> Transfer Fcn11/1
  Demux6/3 -> Transfer Fcn4/1
  PresIn/1 -> Demux6/1
  Demux6/4 -> Transfer Fcn5/1
  Transfer Fcn5/1 -> Sum3/1
  Mux21/1 -> PresOut/1
  Demux6/1 -> Transfer Fcn3/1
  Transfer Fcn6/1 -> Sum4/1
  Transfer Fcn4/1 -> Sum2/1
  Demux6/6 -> Transfer Fcn7/1
  Transfer Fcn2/1 -> Sum1/1
  Transfer Fcn8/1 -> Sum6/1
  Transfer Fcn9/1 -> Sum7/1
  Transfer Fcn11/1 -> Sum9/1
  Transfer Fcn3/1 -> Sum/1
  Transfer Fcn10/1 -> Sum8/1
  Demux6/2 -> Transfer Fcn2/1
  Demux6/8 -> Transfer Fcn9/1
  Demux6/9 -> Transfer Fcn10/1
  Demux6/7 -> Transfer Fcn8/1
  Demux6/5 -> Transfer Fcn6/1
  Transfer Fcn7/1 -> Sum5/1
  Sum/1 -> Mux21/1
  Sum1/1 -> Mux21/2
  Sum2/1 -> Mux21/3
  Sum3/1 -> Mux21/4
  Sum4/1 -> Mux21/5
  Sum5/1 -> Mux21/6
  Sum6/1 -> Mux21/7
  Sum7/1 -> Mux21/8
  Sum8/1 -> Mux21/9
  Sum9/1 -> Mux21/10
  Clock/1 -> 1-D Lookup Table/1
  PresDecel/1 -> Transfer Fcn1/1
  1-D Lookup Table/1 -> ?
  Transfer Fcn1/1 -> Sum9/2, Sum8/2, Sum7/2, Sum/2, Sum1/2, Sum2/2, Sum3/2, Sum4/2, Sum5/2, Sum6/2

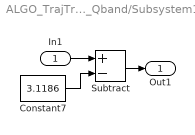
== system ALGO_TrajTrack_Qband/Subsystem1 ==
  In1 : Inport
  Constant7 : Constant  Value=3.1186
  Subtract : Sum  Inputs=+-
  Out1 : Outport
  wires:
  Constant7/1 -> Subtract/2
  In1/1 -> Subtract/1
  Subtract/1 -> Out1/1

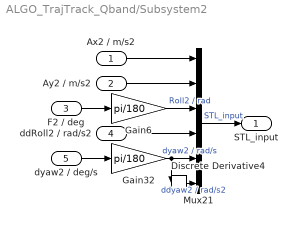
== system ALGO_TrajTrack_Qband/Subsystem2 ==
  Ax2 / m/s2 : Inport
  Ay2 / m/s2 : Inport  Port=2
  F2 / deg : Inport  Port=3
  ddRoll2 / rad/s2 : Inport  Port=4
  dyaw2 / deg/s : Inport  Port=5
  Discrete Derivative4 : simulink/Discrete/Discrete Derivative  gainval=1.0  ICPrevScaledInput=0.0  OutMin=[]  OutMax=[]  OutDataType=fixdt(1, 16)  OutScaling=2^-10  DoSatur=off
  Gain32 : Gain  Gain=pi/180
  Gain6 : Gain  Gain=pi/180
  Mux21 : Mux  Inputs=6
  STL_input : Outport
  wires:
  Gain6/1 -> Mux21/3  "Roll2 / rad"
  Ax2 / m/s2/1 -> Mux21/1
  Discrete Derivative4/1 -> Mux21/6  "ddyaw2 / rad/s2"
  Gain32/1 -> Discrete Derivative4/1, Mux21/5  "dyaw2 / rad/s"
  dyaw2 / deg/s/1 -> Gain32/1
  F2 / deg/1 -> Gain6/1
  Mux21/1 -> STL_input/1  "STL_input"
  Ay2 / m/s2/1 -> Mux21/2
  ddRoll2 / rad/s2/1 -> Mux21/4

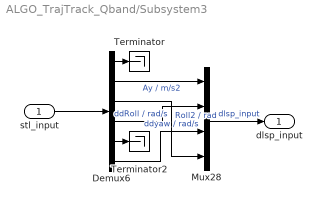
== system ALGO_TrajTrack_Qband/Subsystem3 ==
  stl_input : Inport
  Demux6 : Demux  Outputs=6
  Mux28 : Mux
  Terminator : Terminator
  Terminator2 : Terminator
  dlsp_input : Outport
  wires:
  Demux6/6 -> Mux28/3  "ddyaw / rad/s"
  Demux6/4 -> Mux28/2  "ddRoll / rad/s"
  stl_input/1 -> Demux6/1
  Demux6/3 -> Mux28/4  "Roll2 / rad"
  Mux28/1 -> dlsp_input/1  "dlsp_input"
  Demux6/1 -> Terminator/1
  Demux6/2 -> Mux28/1  "Ay / m/s2"
  Demux6/5 -> Terminator2/1

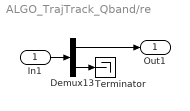
== system ALGO_TrajTrack_Qband/re ==
  In1 : Inport
  Demux13 : Demux  Outputs=2
  Terminator : Terminator
  Out1 : Outport
  wires:
  Demux13/2 -> Terminator/1
  In1/1 -> Demux13/1
  Demux13/1 -> Out1/1

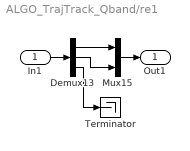
== system ALGO_TrajTrack_Qband/re1 ==
  In1 : Inport
  Demux13 : Demux  Outputs=3
  Mux15 : Mux  Inputs=2
  Terminator : Terminator
  Out1 : Outport
  wires:
  Mux15/1 -> Out1/1
  In1/1 -> Demux13/1
  Demux13/2 -> Mux15/2
  Demux13/1 -> Mux15/1
  Demux13/3 -> Terminator/1

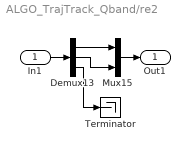
== system ALGO_TrajTrack_Qband/re2 ==
  In1 : Inport
  Demux13 : Demux  Outputs=3
  Mux15 : Mux  Inputs=2
  Terminator : Terminator
  Out1 : Outport
  wires:
  Demux13/3 -> Terminator/1
  Demux13/1 -> Mux15/1
  Demux13/2 -> Mux15/2
  In1/1 -> Demux13/1
  Mux15/1 -> Out1/1

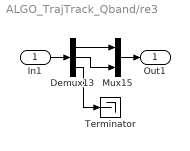
== system ALGO_TrajTrack_Qband/re3 ==
  In1 : Inport
  Demux13 : Demux  Outputs=3
  Mux15 : Mux  Inputs=2
  Terminator : Terminator
  Out1 : Outport
  wires:
  Mux15/1 -> Out1/1
  In1/1 -> Demux13/1
  Demux13/2 -> Mux15/2
  Demux13/1 -> Mux15/1
  Demux13/3 -> Terminator/1

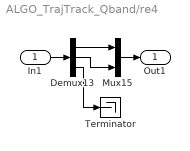
== system ALGO_TrajTrack_Qband/re4 ==
  In1 : Inport
  Demux13 : Demux  Outputs=3
  Mux15 : Mux  Inputs=2
  Terminator : Terminator
  Out1 : Outport
  wires:
  Demux13/3 -> Terminator/1
  Demux13/1 -> Mux15/1
  Demux13/2 -> Mux15/2
  In1/1 -> Demux13/1
  Mux15/1 -> Out1/1

== system ALGO_TrajTrack_Qband/re5 ==
  In1 : Inport
  Demux13 : Demux  Outputs=2
  Terminator : Terminator
  Out1 : Outport
  wires:
  Demux13/1 -> Out1/1
  In1/1 -> Demux13/1
  Demux13/2 -> Terminator/1

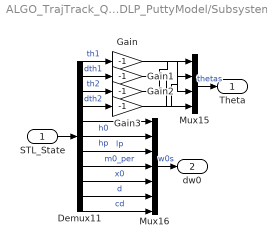
== system ALGO_TrajTrack_Qband/STL2DLP_PuttyModel/Subsystem1 ==
  STL_State : Inport
  Demux11 : Demux  Outputs=11
  Gain{,1..3} (4 alike) : Gain  Gain=-1
  Mux15 : Mux
  Mux16 : Mux  Inputs=7
  Theta : Outport
  dw0 : Outport  Port=2
  wires:
  Demux11/11 -> Mux16/7  "cd"
  Demux11/10 -> Mux16/6  "d"
  Demux11/5 -> Mux16/1  "h0"
  Demux11/2 -> Gain1/1  "dth1"
  Demux11/9 -> Mux16/5  "x0"
  Mux16/1 -> dw0/1  "w0s"
  Demux11/8 -> Mux16/4  "m0_per"
  Demux11/7 -> Mux16/3  "lp"
  Demux11/6 -> Mux16/2  "hp"
  Demux11/3 -> Gain2/1  "th2"
  Demux11/1 -> Gain/1  "th1"
  Demux11/4 -> Gain3/1  "dth2"
  STL_State/1 -> Demux11/1
  Mux15/1 -> Theta/1  "thetas"
  Gain/1 -> Mux15/3
  Gain1/1 -> Mux15/4
  Gain2/1 -> Mux15/1
  Gain3/1 -> Mux15/2

== matlab function ALGO_TrajTrack_Qband/SP_Model ==
  data: ddy input; ExForce output; ddF input; Theta output
function [ExForce,Theta] = SP_Model(ddy,ddF)
persistent sim_param Ts y0
%% 定义摆
if isempty(Ts)
%SP模型，共5个参数拟合
% 参数 m1 h0 hp lp coeff
x=[10890,1.5,0.13,0.97,0.13];
% 获取参数
sim_param=getParam_SP(x);
%初始状态量
y0=zeros(9,1);
%采样时间
Ts=0.005;
end

y=y0;

%% 求解微分方程
dy=zeros(9,1);
dy(1)=y(2);
dy(2)=ddy;
dy(3)=(dy(2)-y(3))/Ts;
dy(4)=y(5);
dy(5)=ddF;
dy(6)=(dy(5)-y(6))/Ts;
dy(7)=y(8);
dy(8)=calc_ddth_SP(y,sim_param);
dy(9)=(dy(8)-y(9))/Ts;
y=y0+dy*Ts;
%% 计算三向力输出
[Fy,Fz,Mx]=calc_Fp_SP(y,sim_param);
ExForce=[Fy,Fz,Mx];
%% 更新状态量
y0=y;
th=y(7);
dth=y(8);
Theta=[th,dth];
end

%% 根据变量获取参数
function sim_param=getParam_SP(x)
%根据变量生成传输参数
TotMass=14462;
m1=x(1);%参数1
m0=TotMass-m1;
h0=x(2);%参数2
hp=x(3);%参数3
lp=x(4);%参数4
g=9.806;
coeff=x(5);%参数5
sim_param=[m0,m1,h0,hp,lp,g,coeff];
end

%% 求解三向力输出
function [Fy,Fz,Mx] = calc_Fp_SP(state,param)
% sim_param=[m0,m1,h0,hp,lp,g,coeff];
m0=param(1);
m1=param(2);
h0=param(3);
hp=param(4);
lp=param(5);
g=param(6);
% co=param(7);

% y=state(1);
% dy=state(2);
ddy=state(3);
f=state(4);
df=state(5);
ddf=state(6);
th=state(7);
dth=state(8);
ddth=state(9);

%定义运算符简写
sf=sin(f);
cf=cos(f);
s2=sin(th+f);
c2=cos(th+f);
L=lp+hp;
%定义质量块的 位置矢量
exh=0.77; %额外增加的高度是罐底到车轴心的高度
R0=[-(exh+h0)*sf,(exh+h0)*cf];

R1=[-(exh+L)*sf+lp*s2
    (exh+L)*cf-lp*c2];

ddRp0=[ddy-h0*cf*ddf+df^2*h0*sf
-h0*sf*ddf-h0*cf*df^2+g];

ddRp1=[ddy+ddf*(-L*cf+lp*c2)+ddth*(lp*c2)+df^2*(L*sf-lp*s2)+dth^2*(-lp*s2)+df*dth*(-2*lp*s2)
ddf*(-L*sf+lp*s2)+ddth*(lp*s2)+df^2*(-L*cf+lp*c2)+dth^2*(lp*c2)+df*dth*(2*lp*c2)+g];

Fp=m0*ddRp0+m1*ddRp1;
Fy=Fp(1)*cf-(-Fp(2))*sf;
Fz=(-Fp(2))*cf+Fp(1)*sf;
Mx0=(m0*(R0(1)*-ddRp0(2)+R0(2)*ddRp0(1)));
Mx1=(m1*(R1(1)*-ddRp1(2)+R1(2)*ddRp1(1)));

Mx=Mx0+Mx1;

end
%% 求解ddth
function ddth = calc_ddth_SP(state,param)
% sim_param=[m0,m1,h0,hp,lp,g,coeff];
% m0=param(1);
% m1=param(2);
% h0=param(3);
hp=param(4);
lp=param(5);
g=param(6);
co=param(7);

% y=state(1);
% dy=state(2);
ddy=state(3);
f=state(4);
df=state(5);
ddf=state(6);
th=state(7);
dth=state(8);
% ddth=state(9);


%定义运算符简写
s1=sin(th);
c1=cos(th);
s2=sin(th+f);
c2=cos(th+f);
L=lp+hp;

ddth=-(ddy*lp*c2+ddf*(-lp*L*c1+lp^2)-df^2*lp*L*s1+g*lp*s2)/(lp^2);
ddth=ddth-co*dth;

end

== matlab function ALGO_TrajTrack_Qband/LTR_calc  ==
  data: TireFz input; LTR output
function LTR = fcn(TireFz)
% 分配物理量
FzL=sum(TireFz(1:5));
FzR=sum(TireFz(6:10));
% 进行计算
LTR=(FzL-FzR)/(FzL+FzR);
end

== matlab function ALGO_TrajTrack_Qband/STL_Model_50per ==
  data: STL_input input; GenForce output; basin1_pos output; basin2_pos output; surf_pos output; basin1_v output; basin2_v output; surf_v output; dev output; STL_state_vec output
%% 函数：滑动天平模型非线性状态转移函数
% 采用x(k+1) = f(x(k),u(k))的方式改写STL模型，以用于其线性化的实施
% 可以选择按照dx = f(x,u)的方式来改写STL模型
%%% 输入：tspan [t0 tf]
%         Ts    采样时间
%         u     [ax;      01
%                ay;      02
%                droll;   03
%                droll;   04
%                ddroll;  05
%                ddyaw]   06
%         Params 
%                ka 范数的阶数       01
%                ke 方形系数         02
%                kx x坐标轴的范围    03
%                ky y坐标轴的范围    04
%                kz z坐标轴的范围    05
%                h  曲面底部的静高   06
%                ap 曲线的半长轴     07
%                bp 曲线的半短轴     08 
%                pr 曲线的幂次       09
%                m  晃动部分质量     10
%              damp 小球晃动的阻尼   11
%             xdamp 浴盆x向移动阻尼  12
%              adec 加速度换算系数   13
%           dev_def 静态偏置距离     14 
%             vxdec x方向速度衰减    15
%             axpow 加速度衰减系数   16
%             dev_a dev自衰减系数    17
%             dev_b dev输入系数      18
%        
%  
function [GenForce,basin1_pos,basin2_pos,surf_pos,basin1_v,basin2_v,surf_v,dev,STL_state_vec]  = SlidingLibra_Fun(STL_input)% ddx,ddy,roll,ddf,dth,ddth
    % 初始化输出状态量
    persistent STL_state Params Ts
    if isempty(Ts)
        Ts = 0.01; % 采样时间
        STL_state.x0 = 0;% 初始化状态变量
        STL_state.dx0 = 0;
        STL_state.x1 = 0;
        STL_state.dx1 = 0;
        STL_state.y1 = 0;
        STL_state.dy1 = 0;
        STL_state.x2 = 0;
        STL_state.dx2 = 0;
        STL_state.y2 = 0;
        STL_state.dy2 = 0;
        STL_state.dev = 0;
        STL_state.basin1_pos = [0,0,0];
        STL_state.basin2_pos = [0,0,0];
        STL_state.basin1_v = [0,0,0];
        STL_state.basin2_v = [0,0,0];
        STL_state.surf_pos = [0,0];
        STL_state.surf_v = [0,0];
%         Params 
%                ka 范数的阶数       01
%                ke 方形系数         02
%                kx x坐标轴的范围    03
%                ky y坐标轴的范围    04
%                kz z坐标轴的范围    05
%                h  曲面底部的静高   06
%                ap 曲线的半长轴     07
%                bp 曲线的半短轴     08 
%                pr 曲线的幂次       09
%                m  晃动部分质量     10
%              damp 小球晃动的阻尼   11
%             xdamp 浴盆x向移动阻尼  12
%              adec 加速度换算系数   13
%               dev 偏置距离         14 
%             vxdec x方向速度衰减    15
%             axpow 加速度衰减系数   16
%             dev_a dev自衰减系数    17
%             dev_b dev输入系数      18
        Params = [3.593, 7.7146, 1.0424, 1.2903, 3.2396, 1.2631, ...
            15.5018, 0.6069, 0.53091, 14498.6641, 0.17393, 3.8431, ...
            0.55681, 3.1186, 9.1364, 0.42295, 20.1983, 0.1208];
        exh = 0.77;
        Params(11) = 0.5;
        Params(6) = Params(6) + exh;

    end
    STL_input(abs(STL_input)>20) = 0;
    ddx = -STL_input(1); % ddx是车辆受到的，但是转换为液体受到的，就要加个负号
    ddy = -STL_input(2); % ddy是车辆受到的，但是转换为液体受到的，就要加个负号
    roll = STL_input(3);
    ddf = -STL_input(4);  % ddf是车辆受到的，但是转换为液体受到的，就要加个负号
    dth = STL_input(5);
    ddth = STL_input(6); % ddth是车辆受到的，但是转换为液体受到的，就要加个负号

    %% 2D计算程序
    %% 仿真参数设置
    % 时间与绘图设置
    Eps = 1e-5; % 数值求导的微小步长

    % 设置曲面方程
    surf4lm = Surface4LumpedMass(Params(1),Params(2),Params(3),Params(4),Params(5),Params(6));
    Surface = @(x)surf4lm.Value(x);

    
    % 设置曲线方程
    ap = Params(7);
    bp = Params(8);
    pr = Params(9);
    Curve = @(x) real(sign(-bp*(1-x.*x/(ap*ap)))*abs(-bp*(1-x.*x/(ap*ap))).^(1/pr)).*sign(ap-abs(x));
    
    % 设置物理属性
    m = Params(10)/2;     % kg 单个小球质量
    damp = Params(11);    %   曲面内晃动阻尼系数
    xdamp = Params(12);   %   曲面沿x方向滑动阻尼系数
    adec = Params(13);    %   加速度换算系数
    dev0 = Params(14);    %   偏置距离
    vxdec = Params(15);
    damp = [vxdec*damp, damp, (1+vxdec)*damp/2];
    axpow = Params(16);
    dev_a = Params(17);
    dev_b = Params(18);
    
    %% 初始状态设置
    basin1_pos = [STL_state.x1,STL_state.y1,Surface([STL_state.x1,STL_state.y1])];% 第一个球
    basin1_v = STL_state.basin1_v; % 第一个球的速度
    basin2_pos = [STL_state.x2,STL_state.y2,Surface([STL_state.x2,STL_state.y2])];% 第二个球
    basin2_v = STL_state.basin2_v; % 第二个球的速度
    surf_pos = [STL_state.x0, Curve(STL_state.x0)]; % 滑动浴盆的位置
    surf_v = STL_state.surf_v; % 滑动浴盆的速度
    dev = dev0 + STL_state.dev;
    
    %% 定义输入量
    a =  [ddx;ddy;-9.806];  % az
    f = roll;
        

    %% 更新曲面的滑动
    %计算当前位置的曲线斜率
    surfGrad=NumGrad(Curve,surf_pos(1),Eps);
    surfGradVec=[1,surfGrad];
    theta=atan(surfGrad);
    %计算曲线姿态
    ax=(sign(a(1))*abs(a(1))^axpow)*adec;
    az=a(3);
    a__=[ax,az]';
    %计算无阻碍时的新位置
    pos0_=surf_pos+surf_v*Ts+1/2*a__'*Ts*Ts;
    move0_=pos0_-surf_pos;
    dist0=norm(move0_);
    %计算有阻挡时的位置更新
    dtheta=sign(dot([surfGrad,-1],move0_))*acos(dot(surfGradVec,move0_)/(norm(surfGradVec)*dist0));
    newPosx_=pos0_(1)-dist0*sin(theta)*sin(dtheta);
    pos0_=surf_pos;
    surf_pos=[newPosx_,Curve(newPosx_)];
    %根据位移差距计算当前速度
    move_=surf_pos-pos0_;
    surf_v=[move_(1)/Ts,move_(2)/Ts]*(1-Ts*xdamp);

    %% 更新两个浴盆的分离（dev变化）
    dev = dev0 + (1-dev_a*Ts)*(dev-dev0) + (dev_b*Ts)*abs(dth);

    %% 更新集中质量1相对曲面的摆动
    % 计算当前位置的曲面梯度
    Grad=NumGrad(Surface,basin1_pos(1:2)',Eps);
    NormVec=[Grad',-1];
    % 计算曲面姿态
    ax=a(1);ay=a(2);az=a(3);
    posx=basin1_pos(1)+surf_pos(1)+dev;
    posy=basin1_pos(2);
    posz=basin1_pos(3)+surf_pos(2);
    a_=[ax                   - ddth*posy;...
       (ay*cos(f)-az*sin(f)) + ddth*posx - ddf*posz;...
       (az*cos(f)+ay*sin(f)) + ddf*posy];
    %计算无阻碍时的新位置
    pos0=basin1_pos+basin1_v*Ts+1/2*a_'*Ts*Ts;
    move0=pos0-basin1_pos;
    %计算有阻挡时的位置更新
    proj=move0-dot(move0,NormVec)*NormVec/norm(NormVec);
    newPosx=basin1_pos(1)+proj(1);
    newPosy=basin1_pos(2)+proj(2);
    pos0=basin1_pos;
    basin1_pos=[newPosx,newPosy,Surface([newPosx,newPosy])];
    
    %根据位移差距计算当前速度
    move=basin1_pos-pos0;
    v0=basin1_v;
    basin1_v=move/Ts.*(1-Ts*damp);
    %根据速度差计算加速度
    acc=(basin1_v-v0)/Ts;

    %根据加速度计算力
    force1 = -m*(acc-a_');
    %根据力和位置计算力矩
    fx=force1(1);fy=force1(2);fz=force1(3);
    moment1 = [(posy*fz-posz*fy);(posz*fx-posx*fz);(posx*fy-posy*fx)];


    %% 更新集中质量2相对曲面的摆动
    % 计算当前位置的曲面梯度
    Grad=NumGrad(Surface,basin2_pos(1:2)',Eps);
    NormVec=[Grad',-1];
    % 计算曲面姿态
    posx=basin2_pos(1)+surf_pos(1)-dev;
    posy=basin2_pos(2);
    posz=basin2_pos(3)+surf_pos(2);
   
    a_=[ax                   - ddth*posy;...
       (ay*cos(f)-az*sin(f)) + ddth*posx - ddf*posz;...
       (az*cos(f)+ay*sin(f)) + ddf*posy];
    %计算无阻碍时的新位置
    pos0=basin2_pos+basin2_v*Ts+1/2*a_'*Ts*Ts;
    move0=pos0-basin2_pos;
    %计算有阻挡时的位置更新
    proj=move0-dot(move0,NormVec)*NormVec/norm(NormVec);
    newPosx=basin2_pos(1)+proj(1);
    newPosy=basin2_pos(2)+proj(2);
    pos0=basin2_pos;
    basin2_pos=[newPosx,newPosy,Surface([newPosx,newPosy])];
    %根据位移差距计算当前速度
    move=basin2_pos-pos0;
    v0=basin2_v;
    basin2_v=move/Ts.*(1-Ts*damp);
    %根据速度差计算加速度
    acc=(basin2_v-v0)/Ts;

    %根据加速度计算力
    force2 = -m*(acc-a_');
    %根据力和位置计算力矩
    fx=force2(1);fy=force2(2);fz=force2(3);
    moment2 = [(posy*fz-posz*fy);(posz*fx-posx*fz);(posx*fy-posy*fx)];


    %记录数据
    Force=force1'+force2';
    Moment=moment1+moment2;
    
    STL_state.basin1_pos = basin1_pos;
    STL_state.basin2_pos = basin2_pos;
    STL_state.basin1_v = basin1_v;
    STL_state.basin2_v = basin2_v;
    STL_state.dev = dev - dev0;
    STL_state.surf_pos = surf_pos;
    STL_state.surf_v = surf_v;
    STL_state.x0 = surf_pos(1);
    STL_state.x1 = basin1_pos(1);
    STL_state.x2 = basin2_pos(1);
    STL_state.y1 = basin1_pos(2);
    STL_state.y2 = basin2_pos(2);
    STL_state_vec = [surf_pos(1); surf_v(1); ...
        basin1_pos(1); basin1_pos(2); basin1_v(1); basin1_v(2); ...
        basin2_pos(1); basin2_pos(2); basin1_v(1); basin1_v(2); dev - dev0]';
    GenForce = [Force;Moment]';
end

== matlab function ALGO_TrajTrack_Qband/DLSP_Model_50per ==
  data: GenForce output; DLSP_input input; Theta_in input; Theta output; dParams input
%% 函数：双摆线性状态转移函数
%%% 输入：Theta0 初始状态，[th1 dth1 th2 dth2]
%         Ts    采样时间
%         DLSP_input 输入量，[ay,ddroll,ddyaw,roll]
%         Params Dual-LSP模型的参数共7个
%                h0 m0距侧倾中心高度 01
%                hp mp距侧倾中心高度 02
%                lp mp的摆长         03
%                m0 m0的质量大小     04
%                x0 两摆前移距离     05
%                d  两摆半分离距     06
%                cd 摆动阻尼         07
%
%%% 输出：GenForce 输出力，3维向量分别为Fy Mx Mz
%        Theta 下一个时刻的状态，同样为[th1 dth1 th2 dth2]
%

function [GenForce,Theta] = DualLSP_Fcn(DLSP_input,Theta_in,dParams)
    persistent Ts ParamsDLSP coeff_theta coeff_params
    persistent Theta0
    if isempty(Ts)
        Theta0 = zeros(4,1);
        Ts = 0.01;
        coeff_theta = 0.9;
        coeff_params = 0.9;
        % ParamsDLSP = [1.5, 0.13, 0.77, 0.4763, 0.0, 3.5, 0.53];
        ParamsDLSP = [1.5, 0.13, 0.77, 0.4763, 0.0, 3.5, 0.33];
        exh = 0.77;
        ParamsDLSP(1:2) = ParamsDLSP(1:2) + exh;
    end
    % 获取Dual-LSP模型参数

    [h0,hp,lp,m0,mp,x0,d,cd] = Dual_LSP_getParams(ParamsDLSP+coeff_params*dParams'); 
   
    g = 9.806;
    % 获取当期时刻状态量
    Theta0 = (1-coeff_theta)*Theta0+coeff_theta*Theta_in;
    th1 = Theta0(1);
    dth1 = Theta0(2);
    th2 = Theta0(3);
    dth2 = Theta0(4);
    
    % 获取当前时刻输入量
    ddy = DLSP_input(1); 
    ddf = DLSP_input(2);
    ddyaw = DLSP_input(3); 
    f = DLSP_input(4); 


    % 计算当前时刻动力学
    ddy1 = ddy + ddyaw*(x0 + d);
    ddy2 = ddy + ddyaw*(x0 - d);
    x1 = x0 + d;
    x2 = x0 - d;
    ddth1 = -(1/lp*ddy1 + (2-hp/lp)*ddf + g/lp*(f + th1) + cd*dth1);
    ddth2 = -(1/lp*ddy2 + (2-hp/lp)*ddf + g/lp*(f + th2) + cd*dth2);
    dth1 = dth1 + Ts*ddth1;
    dth2 = dth2 + Ts*ddth2;
    th1 = th1 + Ts*dth1;
    th2 = th2 + Ts*dth2;
    Theta = [th1 dth1 th2 dth2]';
    Fy1 = 1/2*(-(mp + m0)*ddy1 + (m0*h0 + mp*hp)*ddf - mp*lp*ddth1);
    Fy2 = 1/2*(-(mp + m0)*ddy2 + (m0*h0 + mp*hp)*ddf - mp*lp*ddth2);
    Fy = Fy1 + Fy2;
    Mx = (m0*h0 + mp*hp)*(ddy + ddyaw*x0) - (m0*h0^2 + mp*hp^2)*ddf ...
        + (m0*h0 + mp*hp)*g*f + mp*hp*lp*(ddth1 + ddth2)/2 - 1/2*mp*lp*g*(th1 + th2);
    Mz = -1/2*((x1 + x2)*(m0 + mp)*ddy - (m0 + mp)*(x1^2 + x2^2)*ddyaw ...
        + (x1 + x2)*(m0*h0 + mp*hp)*ddf - mp*lp*(x2*ddth2 + x1*ddth1));
    
    GenForce = [Fy Mx Mz];

    % 更新存储的状态量
    Theta0 = Theta;
end

function [h0,hp,lp,m0,mp,x0,d,cd] = Dual_LSP_getParams(Params)
    m = 14462; % TotalWeight
    h0 = Params(1);
    hp = Params(2);
    lp = Params(3);
    m0 = m*Params(4);
    mp = m - m0;
    x0 = Params(5);
    d = Params(6);
    cd = Params(7);
end
